simulink model "Wrapper_SOA_demo_codegen"  (R2024b)
settings: Solver=FixedStepAuto  StartTime=0.0  StopTime=10.0  FixedStep=0.2  RelTol=1e-3
undefined symbols (not defined in the file or in its folder): call_a_f
settings Model: Tag=EP_AA_WRAPPER_TOPLEVEL  Creator=nabilekhoury  LastModifiedBy=nabilekhoury
settings OptimizationCC: DefaultParameterBehavior=Inlined  EnhancedBackFolding=on  PassReuseOutputArgsAs=Individual arguments  ZeroExternalMemoryAtStartup=off  ZeroInternalMemoryAtStartup=off  OptimizeBlockOrder=speed  DifferentSizesBufferReuse=on  OptimizationCustomize=off  EfficientTunableParamExpr=on
settings DebuggingCC: ParameterTunabilityLossMsg=error
settings SFSimCC: MATLABDynamicMemAlloc=off  SimTargetLang=C++
settings RTWCC: Description=Embedded Coder  SystemTargetFile=ert.tlc  GenCodeOnly=on  TemplateMakefile=ert_default_tmf  CustomSourceCode="#include \"SOA_demo_codegen_adapter.h\""  CustomInitializer=sut_initialize();  TargetLang=C++  GPUComputeCapability=3.5
settings CodeAppCC: ForceParamTrailComments=on  IgnoreCustomStorageClasses=off  MaxIdLength=256  OperatorAnnotations=on  SimulinkDataObjDesc=on  SFDataObjDesc=on  CustomSymbolStrGlobalVar=w_$R$N$M  CustomSymbolStrType=w_$N$R$M_T  InsertBlockDesc=on
settings ERTTargetCC: TargetLangStandard=C++11 (ISO)  GenerateSampleERTMain=on  RootIOFormat=Structure reference  ERTCustomFileTemplate=example_file_process.tlc  DynamicArrayContainerType=coder::array

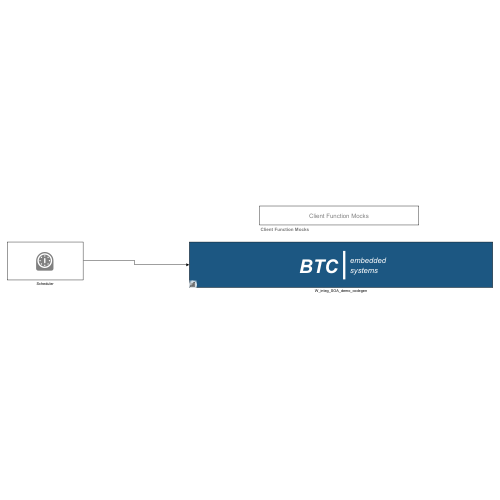
[thumbnail: Simulink's stored preview of the top-level diagram]
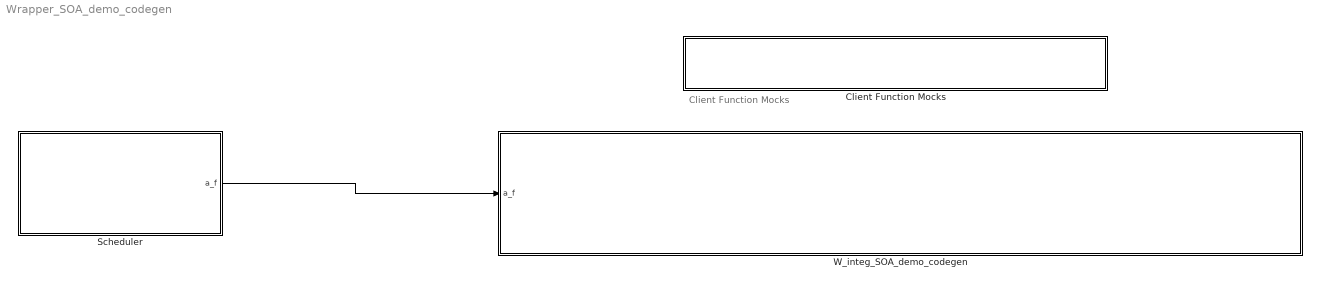
== system Wrapper_SOA_demo_codegen ==
  note: Client Function Mocks
  Client Function Mocks : Subsystem
      mask Display: color('gray'); disp('{\fontsize{16}Client Function Mocks}', 'texmode', 'on');
  Scheduler : Subsystem
      mask Display: disp('\color{gray}\fontsize{50}⏲', 'texmode', 'on');
  W_integ_SOA_demo_codegen : Subsystem  Variant=on  VariantControlMode=label  LabelModeActiveChoice=orig  PropagateVariantConditions=on
      settings: OpenFcn=open_system(gcb, 'mask');
      mask DialogControl DescGroupVar Prompt: BTC Embedded Systems SUT block
      mask DialogControl DescTextVar Prompt: This is the BTC Embedded Systems SUT block, referencing the original Adaptive AUTOSAR model.
      mask DialogControl DescButVar Prompt: Open original model...
      mask DialogControl DescButVar Callback: open_system('SOA_demo_codegen');
      mask Display: disp('\color{white}\it\fontsize{20}                          embedded\newline                          systems', 'texmode', 'on');disp('{{\color{white}\bf\fontsize{50}\it   BTC}  \fontsize{80}|      \color{black}\fontsize{20}\newline }', 'texmode','on');
  wires:
  Scheduler/1(a_f) -> W_integ_SOA_demo_codegen/1(a_f)

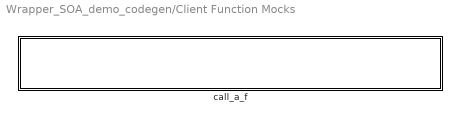
== system Wrapper_SOA_demo_codegen/Client Function Mocks ==
  call_a_f : Subsystem  TreatAsAtomicUnit=on

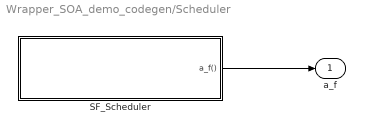
== system Wrapper_SOA_demo_codegen/Scheduler ==
  SF_Scheduler : Stateflow chart  TreatAsAtomicUnit=on
  a_f : Outport
  wires:
  SF_Scheduler/1(a_f()) -> a_f/1

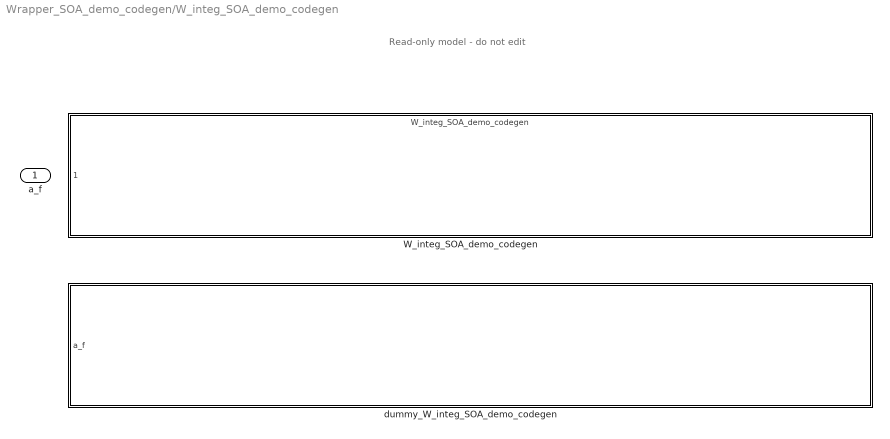
== system Wrapper_SOA_demo_codegen/W_integ_SOA_demo_codegen ==
  note: Read-only model - do not edit
  a_f : Inport
  W_integ_SOA_demo_codegen : ModelReference  Tag=BTC AUTOSAR Main Model Reference Block  ModelNameDialog=W_integ_SOA_demo_codegen  SimulationMode=Normal  ScheduleRates=on  VariantControl=orig  ModelReferenceVersion=1.2
  dummy_W_integ_SOA_demo_codegen : Subsystem  VariantControl=dummy

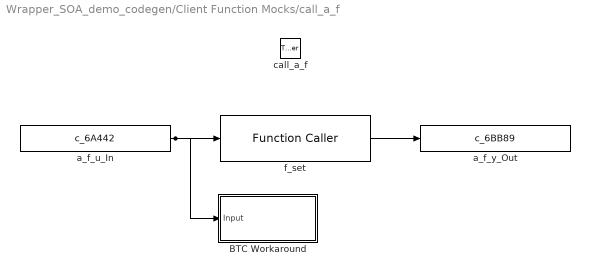
== system Wrapper_SOA_demo_codegen/Client Function Mocks/call_a_f ==
  call_a_f : TriggerPort  TriggerType=function-call  IsSimulinkFunction=on  FunctionName=call_a_f  VariantControl=(inherit)
  BTC Workaround : Subsystem
      settings: OpenFcn=open_system(gcb, 'mask');
      mask DialogControl DescGroupVar Prompt: BTC Embedded Systems MIL stabilizer
      mask DialogControl DescTextVar Prompt: The BTC Embedded Systems MIL stabilizer prevents a known Matlab 2023b issue that results in a crash. It has no effect on the signal. Do not edit its contents.
      mask Display: disp('\color[rgb]{0.11,0.34,0.51}\bf MIL stabilizer', 'texmode', 'on');
  a_f_u_In : DataStoreRead  DataStoreName=c_6A442  IndexOptions=Index vector (dialog)  Indices=1  OutputSizes=1
  a_f_y_Out : DataStoreWrite  DataStoreName=c_6BB89  IndexOptions=Index vector (dialog)  Indices=1  OutputSizes=1
  f_set : FunctionCaller  FunctionPrototype=y = sut_a_f_set(u)  InputArgumentSpecifications=double(0)  OutputArgumentSpecifications=double(0)
  wires:
  a_f_u_In/1 -> f_set/1, BTC Workaround/1(Input)
  f_set/1 -> a_f_y_Out/1

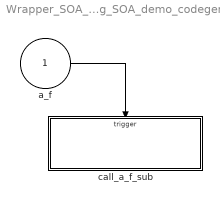
== system Wrapper_SOA_demo_codegen/W_integ_SOA_demo_codegen/dummy_W_integ_SOA_demo_codegen ==
  a_f : Inport  OutputFunctionCall=on
  call_a_f_sub : Subsystem  TreatAsAtomicUnit=on
  wires:
  a_f/1 -> call_a_f_sub/Trigger

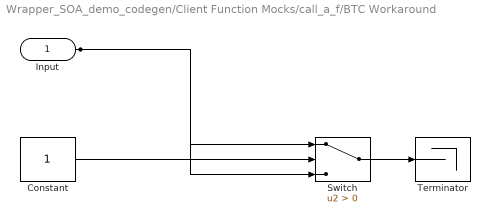
== system Wrapper_SOA_demo_codegen/Client Function Mocks/call_a_f/BTC Workaround ==
  Input : Inport
  Constant : Constant
  Switch : Switch  Criteria=u2 > Threshold  SaturateOnIntegerOverflow=off  InputSameDT=off
  Terminator : Terminator
  wires:
  Input/1 -> Switch/1, Switch/3
  Switch/1 -> Terminator/1
  Constant/1 -> Switch/2

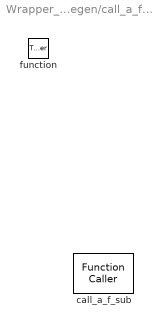
== system Wrapper_SOA_demo_codegen/W_integ_SOA_demo_codegen/dummy_W_integ_SOA_demo_codegen/call_a_f_sub ==
  function : TriggerPort  TriggerType=function-call  VariantControl=(inherit)
  call_a_f_sub : FunctionCaller  FunctionPrototype=call_a_f()  InputArgumentSpecifications=<Enter example>  OutputArgumentSpecifications=<Enter example>

== stateflow chart Wrapper_SOA_demo_codegen/Scheduler/SF_Scheduler ==
  state Schedule
    en:
    send(a_f);
    du:
    on every(1, tick):send(a_f);
  (default) -> Schedule : /*Update the Order/Rate/Asynchronous calls of the runnables*/
  events: a_f output FUNCTION_CALL_EVENT
